simulink model "retificador_controlado"  (R2018a)
settings: Solver=VariableStepAuto  StartTime=0.0  StopTime=0.1  RelTol=1e-3
libraries: nesl_utility x16, fl_lib x14, pe_lib x4
settings Model: Creator=Gabriel  LastModifiedBy=Gabriel

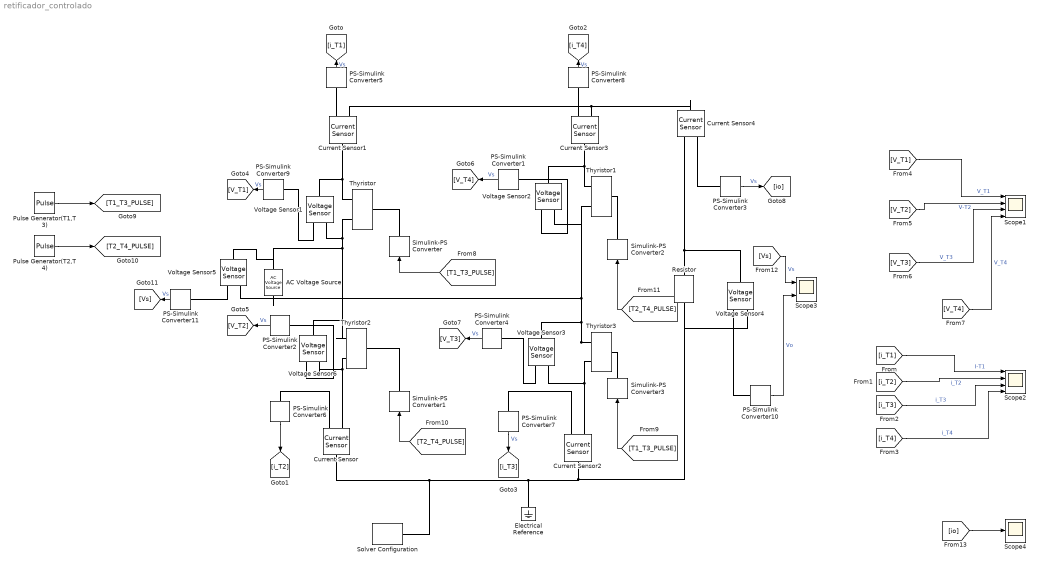
== system retificador_controlado ==
  AC Voltage Source : fl_lib/Electrical/Electrical Sources/AC Voltage Source  amp=250 V  shift=0 deg  frequency=60 Hz  omega=0 rad/s
  Current Sensor{,1..4} (5 alike) : fl_lib/Electrical/Electrical Sensors/Current Sensor
  Electrical Reference : fl_lib/Electrical/Electrical Elements/Electrical Reference
  PS-Simulink Converter{1..9,11} (10 alike) : nesl_utility/PS-Simulink Converter  PhysicalDomain=network_engine_domain  SubClassName=ps_output  LeftPortType=input  RightPortType=output  PseudoPeriodic=off  Frequencies=[]  Unit=1  AffineConversion=off
  PS-Simulink Converter10 : nesl_utility/PS-Simulink Converter  PhysicalDomain=network_engine_domain  SubClassName=ps_output  LeftPortType=input  RightPortType=output  PseudoPeriodic=off  Frequencies=[]  Unit=V  AffineConversion=off
  "Pulse Generator(T1,T3) " : DiscretePulseGenerator  PulseType=Time based  Amplitude=8  Period=1/60  PulseWidth=15000/360  PhaseDelay=1/720
  "Pulse Generator(T2,T4) " : DiscretePulseGenerator  PulseType=Time based  Amplitude=8  Period=1/60  PulseWidth=15000/360  PhaseDelay=21/2160
  Resistor : fl_lib/Electrical/Electrical Elements/Resistor  R=750 Ohm  i_specify=off  i_priority=None  i=0 A  i_nominal_specify=off  i_nominal_unit=A  i_nominal_value=1  v_specify=off  v_priority=None  v=0 V  v_nominal_specify=off  v_nominal_unit=V  v_nominal_value=1
  Scope1 : Scope  NumInputPorts=4
  Scope2 : Scope  NumInputPorts=4
  Scope3 : Scope  NumInputPorts=2
  Scope4 : Scope
  Simulink-PS Converter{,1..3} (4 alike) : nesl_utility/Simulink-PS Converter  PhysicalDomain=network_engine_domain  SubClassName=ps_input  LeftPortType=input  RightPortType=output  PseudoPeriodic=off  Frequencies=[]  NoiseDistribution=none  NoiseParameters=[]  Unit=V  AffineConversion=off  FilteringAndDerivatives=provide  SimscapeFilterOrder=1  InputFilterTimeConstant=0.001  UdotUserProvided=0
  Solver Configuration : nesl_utility/Solver Configuration  PhysicalDomain=network_engine_domain  SubClassName=solver  LeftPortType=input  RightPortType=generic  Tones=[]  Harmonics=[]  SimulateNoise=off  Profile=off  UseLocalSampling=off  EnableSwitchedLinearOptims=on  FrequencyDomain=off  UseCCode=off  RelTol=0.001  AbsTol=1e-06  MinStep=1e-09  ToWorkspace=off  RevertToSquareIcSolve=off  NumHomotopyIterations=100  PhasorMode=off  PhasorModeNumHarmonics=1  DoDC=off  ResidualTolerance=1e-09  UseLocalSolver=off  LocalSolverChoice=NE_BACKWARD_EULER_ADVANCER  LocalSolverSampleTime=0.001  DoFixedCost=off  MaxNonlinIter=3  MaxModeIter=2  LinearAlgebra=Sparse  EquationFormulation=NE_TIME_EF  DelaysMemoryBudget=1024  AutomaticFiltering=on  FilteringTimeConstant=0.001
  Thyristor{,1..3} (4 alike) : pe_lib/Semiconductors/Fundamental Components/Thyristor  Vf=0.8 V  Ron=0.001 Ohm  Goff=1e-5 1/Ohm  Vgt=6 V  Ih=1 A  diode_param=1  diode_Vf=0.8 V  diode_Ron=0.001 Ohm  diode_Goff=1e-5 1/Ohm  diode_C=5e-8 F  diode_iRM=-235 A  diode_iF=300 A  diode_idot=-50 A/us  diode_trr_param=1  diode_trr_factor=3  diode_trr=15 us  diode_Qrr=1.5e+3 s*uA  thermal_loss_option=2  Voff=300 V  Tau=1e-4 s  Tj=[ 298.15 398.15 ] K  Iout_scalar=600 A  Eon_scalar=0.02286 J  Eoff_scalar=0.01714 J  Von_scalar=2.7 V  Iout_data=[ 0 10 50 100 200 400 600 ] A  Eon_data=[ 0 2.9e-4 0.00143 0.00286 0.00571 0.01314 0.02286; 0 5.7e-4 0.00263 0.00514 0.01029 0.02057 0.03029 ] J  Eoff_data=[ 0 2.1e-4 0.00107 0.00214 0.00429 0.009859999999999999 0.01714; 0 4.3e-4 0.00197 0.00386 0.00771 0.01543 0.02271 ] J  Von_data=[ 0 1.1 1.3 1.45 1.75 2.25 2.7; 0 1 1.15 1.35 1.7 2.35 3 ] V
      settings: SourceProductName=Simscape Power Systems  SourceProductBaseCode=PS
  Voltage Sensor{1..6} (6 alike) : fl_lib/Electrical/Electrical Sensors/Voltage Sensor
  wires:
  [i_T1] -> Scope2/1  "I-T1"
  [i_T2] -> Scope2/2  "i_T2"
  [i_T3] -> Scope2/3  "i_T3"
  [i_T4] -> Scope2/4  "i_T4"
  PS-Simulink Converter5/1 -> [i_T1]  "Vs"
  PS-Simulink Converter6/1 -> [i_T2]
  PS-Simulink Converter8/1 -> [i_T4]  "Vs"
  PS-Simulink Converter7/1 -> [i_T3]  "Vs"
  PS-Simulink Converter9/1 -> [V_T1]  "Vs"
  PS-Simulink Converter2/1 -> [V_T2]  "Vs"
  PS-Simulink Converter1/1 -> [V_T4]  "Vs"
  PS-Simulink Converter4/1 -> [V_T3]  "Vs"
  [V_T1] -> Scope1/1  "V_T1"
  [V_T2] -> Scope1/2  "V-T2"
  [V_T3] -> Scope1/3  "V_T3"
  [V_T4] -> Scope1/4  "V_T4"
  PS-Simulink Converter3/1 -> [io]  "Vs"
  "Pulse Generator(T1,T3) "/1 -> [T1_T3_PULSE]
  "Pulse Generator(T2,T4) "/1 -> [T2_T4_PULSE]
  [T1_T3_PULSE] -> Simulink-PS Converter/1
  [T1_T3_PULSE] -> Simulink-PS Converter3/1
  [T2_T4_PULSE] -> Simulink-PS Converter1/1
  [T2_T4_PULSE] -> Simulink-PS Converter2/1
  [io] -> Scope4/1
  PS-Simulink Converter11/1 -> [Vs]  "Vs"
  [Vs] -> Scope3/1  "Vs"
  PS-Simulink Converter10/1 -> Scope3/2  "Vo"
  connections:
  Current Sensor/RConn2 -- Voltage Sensor6/RConn2 -- Thyristor2/RConn1
  Current Sensor2/RConn2 -- Voltage Sensor3/RConn2 -- Thyristor3/RConn1
  Current Sensor3/LConn1 -- Voltage Sensor2/LConn1 -- Thyristor1/RConn2
  Thyristor/RConn2 -- Voltage Sensor1/LConn1 -- Current Sensor1/LConn1
  Thyristor2/RConn2 -- Voltage Sensor6/LConn1 -- Voltage Sensor5/LConn1 -- AC Voltage Source/LConn1 -- Voltage Sensor1/RConn2 -- Thyristor/RConn1
  Current Sensor2/LConn1 -- Voltage Sensor4/RConn2 -- Resistor/RConn1 -- Electrical Reference/LConn1 -- Solver Configuration/RConn1 -- Current Sensor/LConn1
  Current Sensor1/RConn2 -- Current Sensor4/LConn1 -- Current Sensor3/RConn2
  PS-Simulink Converter5/LConn1 -- Current Sensor1/RConn1
  Current Sensor/RConn1 -- PS-Simulink Converter6/LConn1
  PS-Simulink Converter8/LConn1 -- Current Sensor3/RConn1
  PS-Simulink Converter7/LConn1 -- Current Sensor2/RConn1
  Simulink-PS Converter2/RConn1 -- Thyristor1/LConn1
  Simulink-PS Converter/RConn1 -- Thyristor/LConn1
  Simulink-PS Converter1/RConn1 -- Thyristor2/LConn1
  Simulink-PS Converter3/RConn1 -- Thyristor3/LConn1
  PS-Simulink Converter10/LConn1 -- Voltage Sensor4/RConn1
  Thyristor3/RConn2 -- Voltage Sensor3/LConn1 -- Voltage Sensor5/RConn2 -- AC Voltage Source/RConn1 -- Voltage Sensor2/RConn2 -- Thyristor1/RConn1
  Voltage Sensor4/LConn1 -- Resistor/LConn1 -- Current Sensor4/RConn2
  Current Sensor4/RConn1 -- PS-Simulink Converter3/LConn1
  PS-Simulink Converter11/LConn1 -- Voltage Sensor5/RConn1
  Voltage Sensor1/RConn1 -- PS-Simulink Converter9/LConn1
  Voltage Sensor6/RConn1 -- PS-Simulink Converter2/LConn1
  Voltage Sensor3/RConn1 -- PS-Simulink Converter4/LConn1
  Voltage Sensor2/RConn1 -- PS-Simulink Converter1/LConn1
